simulink model "mbd_example_adc"  (R2022b)
settings: Solver=FixedStepDiscrete  StartTime=0.0  StopTime=10.0  RelTol=1e-3  EnableMultiTasking=on
PostLoadFcn:
  | run([bdroot '_init']);
InitFcn:
  | checkModelFolder(true); % Optional
  | run([bdroot '_init']);
values from neighbouring files (symbols this model uses):
  LED1_Hz = 2    [mbd_example_adc_init.m]
  LED2_Hz = 1    [mbd_example_adc_init.m]
  MBDDiag_Comm_Module = [2 3]    [mbd_example_adc_init.m]
  MBDDiag_Comm_Speed = [921600 921600]    [mbd_example_adc_init.m]
  MBDDiag_Comm_Type = [1 1]    [mbd_example_adc_init.m]
  T_s_LED1 = 1/LED1_Hz    (= 0.5)    [mbd_example_adc_init.m]
  T_s_LED2 = 1/LED2_Hz    (= 1)    [mbd_example_adc_init.m]
libraries: MbdLib_PortalDiag x26, MbdLib_Uart x15, MbdLib_SnapDiag x14, MbdLib_Digital x9, MbdLib_Analog x8, MbdLib_Timer x7, MbdLib_Sys x4, MbdLib_Pwm x2, MbdLib_Required x1
(part 1 of 2)
settings Model: Creator=KenYoshioka  LastModifiedBy=KenYoshioka
settings SolverCC: AutoInsertRateTranBlk=on
settings OptimizationCC: DefaultParameterBehavior=Inlined  DefaultUnderspecifiedDataType=single  EnhancedBackFolding=on  BooleansAsBitfields=on  PassReuseOutputArgsAs=Individual arguments  ZeroExternalMemoryAtStartup=off  ZeroInternalMemoryAtStartup=off  OptimizeBlockOrder=speed  DifferentSizesBufferReuse=on  EfficientTunableParamExpr=on
settings DebuggingCC: MultiTaskDSMMsg=none  ParameterTunabilityLossMsg=error
settings HardwareCC: ProdBitPerPointer=32  ProdBitPerSizeT=32  ProdBitPerPtrDiffT=32  ProdLargestAtomicInteger=Long  ProdLargestAtomicFloat=Double  ProdWordSize=32  ProdHWDeviceType=ARM Compatible->ARM Cortex-M
settings ModelReferenceCC: EnableRefExpFcnMdlSchedulingChecks=on  ModelReferenceNumInstancesAllowed=Single
settings SFSimCC: MATLABDynamicMemAlloc=off
settings RTWCC: Description=MBD Embedded Target STM32 Cortex M4 (real-time)  SystemTargetFile=MBD_STM32_stf.tlc  TemplateMakefile=MBD_STM32.tmf  Toolchain=arm-none-eabi - v10.3
settings CodeAppCC: ForceParamTrailComments=on  IgnoreCustomStorageClasses=off  MaxIdLength=255  OperatorAnnotations=on  SimulinkDataObjDesc=on  SFDataObjDesc=on  InsertBlockDesc=on
settings STFCustomTargetCC: MultiwordLength=256  IncludeMdlTerminateFcn=off  CombineOutputUpdateFcns=on  CombineSignalStateStructs=on  SuppressErrorStatus=on  ERTCustomFileBanners=on  SupportContinuousTime=off  RemoveResetFunc=on  MATLABClassNameForMDSCustomization=Simulink.SoftwareTarget.ERTCustomization  UseToolchainInfoCompliant=on  SystemTargetFile=MBD_STM32_stf.tlc
settings ERTTargetCC: ParMdlRefBuildCompliant=off  CompOptLevelCompliant=off  ConcurrentExecutionCompliant=off  IncludeMdlTerminateFcn=off  CombineSignalStateStructs=on  SuppressErrorStatus=on  SupportNonInlinedSFcns=on  ModelStepFunctionPrototypeControlCompliant=off  CPPClassGenCompliant=off  ExtModeStaticAllocSize=2000  InlinedParameterPlacement=NonHierarchical  ERTCustomFileTemplate=mbd_lib_interface.tlc  MaxLineWidth=110

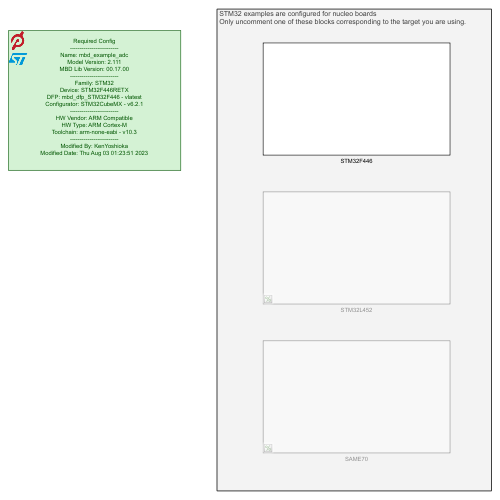
[thumbnail: Simulink's stored preview of the top-level diagram]
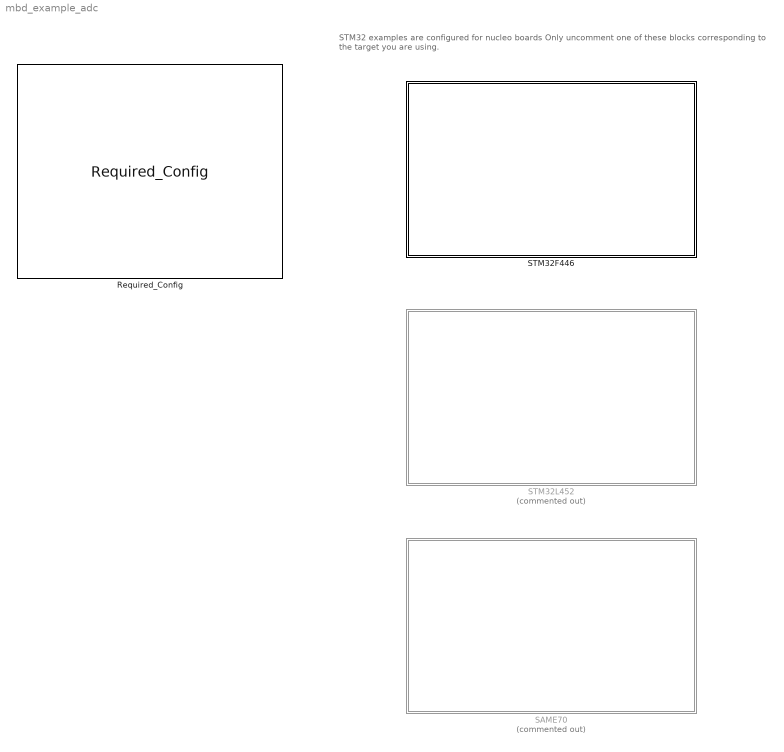
== system mbd_example_adc ==
  note: STM32 examples are configured for nucleo boards
      | Only uncomment one of these blocks corresponding to the target you are using.
  Required_Config : MbdLib_Required/Required_Config  Tag=MBD_Target_Info  Param_update=1
      settings: SourceProductName=Peloton Interface Library
  SAME70 : Subsystem  Commented=on
  STM32F446 : Subsystem
  STM32L452 : Subsystem  Commented=on

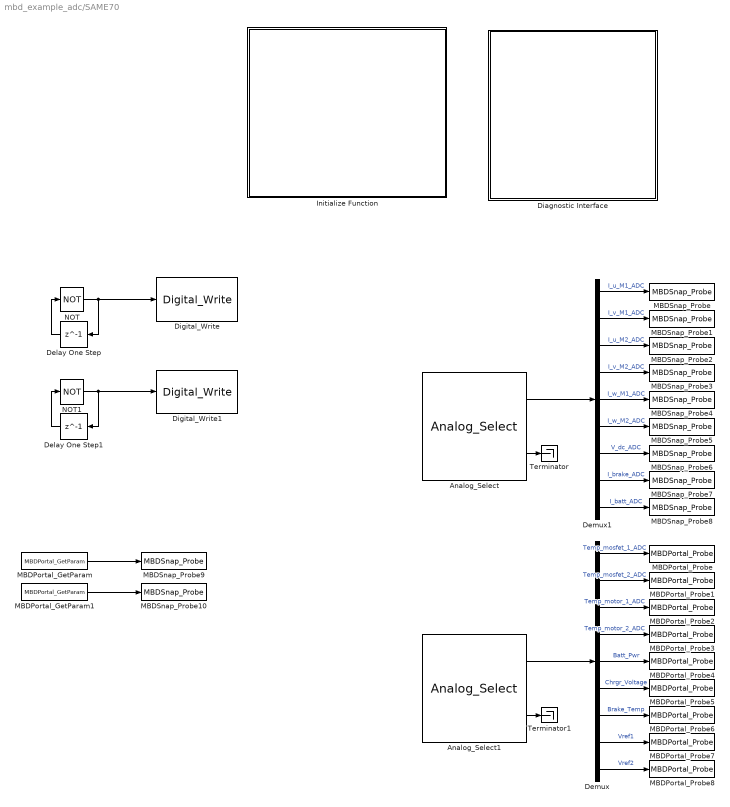
== system mbd_example_adc/SAME70 ==
  Analog_Select : MbdLib_Analog/Analog_Select  Param_triggerMode=No trigger  Param_module=0  Param_timeout=0  Param_outputNum=9  Param_module1=0  Param_index1=0  Param_module2=0  Param_index2=1  Param_module3=0  Param_index3=2  Param_module4=0  Param_index4=3  Param_module5=0  Param_index5=4  Param_module6=0  Param_index6=5  Param_module7=0  Param_index7=6  Param_module8=0  Param_index8=7  Param_module9=0  Param_index9=8  Param_module10=0  Param_index10=9  Param_module11=0  Param_index11=10  Param_module12=0  Param_index12=11  Param_sampleTime=T_s  Param_MBDUpdate=1
      settings: SourceProductName=Peloton Interface Library
  Analog_Select1 : MbdLib_Analog/Analog_Select  Param_triggerMode=No trigger  Param_module=0  Param_timeout=0  Param_outputNum=9  Param_module1=0  Param_index1=0  Param_module2=0  Param_index2=1  Param_module3=0  Param_index3=2  Param_module4=0  Param_index4=3  Param_module5=0  Param_index5=4  Param_module6=0  Param_index6=5  Param_module7=0  Param_index7=6  Param_module8=0  Param_index8=7  Param_module9=0  Param_index9=8  Param_module10=0  Param_index10=9  Param_module11=0  Param_index11=10  Param_module12=0  Param_index12=11  Param_sampleTime=T_s_COMM  Param_MBDUpdate=1
      settings: SourceProductName=Peloton Interface Library
  Delay One Step : Delay  DelayLength=1  SampleTime=LED1_Hz
  Delay One Step1 : Delay  DelayLength=1  SampleTime=LED2_Hz
  Demux : Demux  Outputs=9
  Demux1 : Demux  Outputs=9
  Diagnostic Interface : Subsystem
  Digital_Write : MbdLib_Digital/Digital_Write  Param_module=D  Param_ch=7  Param_sampleTime=-1
      settings: SourceProductName=Peloton Interface Library
  Digital_Write1 : MbdLib_Digital/Digital_Write  Param_module=D  Param_ch=8  Param_sampleTime=-1
      settings: SourceProductName=Peloton Interface Library
  Initialize Function : Subsystem  TreatAsAtomicUnit=on
  MBDPortal_GetParam : MbdLib_PortalDiag/MBDPortal_GetParam  Param_ParamName=start_snapshot  Param_ParamDefault=0  Param_ParamIndex=0  Param_ParamMax=MBDPortal_ParamNum
      settings: SourceProductName=Peloton Component Library
  MBDPortal_GetParam1 : MbdLib_PortalDiag/MBDPortal_GetParam  Param_ParamName=stop_snapshot  Param_ParamDefault=0  Param_ParamIndex=0  Param_ParamMax=MBDPortal_ParamNum
      settings: SourceProductName=Peloton Component Library
  MBDPortal_Probe : MbdLib_PortalDiag/MBDPortal_Probe  Param_SigNameInherited=on  Param_SigName=Temp_mosfet_1_ADC  Param_SigIndex=0  Param_SigMax=MBDPortal_SignalNum  Param_SampleTime=MBDPortal_CommonSampleRate
      settings: SourceProductName=Peloton Component Library
  MBDPortal_Probe1 : MbdLib_PortalDiag/MBDPortal_Probe  Param_SigNameInherited=on  Param_SigName=Temp_mosfet_2_ADC  Param_SigIndex=0  Param_SigMax=MBDPortal_SignalNum  Param_SampleTime=MBDPortal_CommonSampleRate
      settings: SourceProductName=Peloton Component Library
  MBDPortal_Probe2 : MbdLib_PortalDiag/MBDPortal_Probe  Param_SigNameInherited=on  Param_SigName=Temp_motor_1_ADC  Param_SigIndex=0  Param_SigMax=MBDPortal_SignalNum  Param_SampleTime=MBDPortal_CommonSampleRate
      settings: SourceProductName=Peloton Component Library
  MBDPortal_Probe3 : MbdLib_PortalDiag/MBDPortal_Probe  Param_SigNameInherited=on  Param_SigName=Temp_motor_2_ADC  Param_SigIndex=0  Param_SigMax=MBDPortal_SignalNum  Param_SampleTime=MBDPortal_CommonSampleRate
      settings: SourceProductName=Peloton Component Library
  MBDPortal_Probe4 : MbdLib_PortalDiag/MBDPortal_Probe  Param_SigNameInherited=on  Param_SigName=Batt_Pwr  Param_SigIndex=0  Param_SigMax=MBDPortal_SignalNum  Param_SampleTime=MBDPortal_CommonSampleRate
      settings: SourceProductName=Peloton Component Library
  MBDPortal_Probe5 : MbdLib_PortalDiag/MBDPortal_Probe  Param_SigNameInherited=on  Param_SigName=Chrgr_Voltage  Param_SigIndex=0  Param_SigMax=MBDPortal_SignalNum  Param_SampleTime=MBDPortal_CommonSampleRate
      settings: SourceProductName=Peloton Component Library
  MBDPortal_Probe6 : MbdLib_PortalDiag/MBDPortal_Probe  Param_SigNameInherited=on  Param_SigName=Brake_Temp  Param_SigIndex=0  Param_SigMax=MBDPortal_SignalNum  Param_SampleTime=MBDPortal_CommonSampleRate
      settings: SourceProductName=Peloton Component Library
  MBDPortal_Probe7 : MbdLib_PortalDiag/MBDPortal_Probe  Param_SigNameInherited=on  Param_SigName=Vref1  Param_SigIndex=0  Param_SigMax=MBDPortal_SignalNum  Param_SampleTime=MBDPortal_CommonSampleRate
      settings: SourceProductName=Peloton Component Library
  MBDPortal_Probe8 : MbdLib_PortalDiag/MBDPortal_Probe  Param_SigNameInherited=on  Param_SigName=Vref2  Param_SigIndex=0  Param_SigMax=MBDPortal_SignalNum  Param_SampleTime=MBDPortal_CommonSampleRate
      settings: SourceProductName=Peloton Component Library
  MBDSnap_Probe : MbdLib_SnapDiag/MBDSnap_Probe  Param_SigNameInherited=on  Param_SigName=I_u_M1_ADC  Param_SigIndex=0  Param_SigMax=MBDSnap_SignalNum  Param_StartEnable=off  Param_StartOpr=>  Param_StartThr=0  Param_StopEnable=off  Param_StopOpr=>  Param_StopThr=0  Param_StopPost=0  Param_SampleTime=MBDSnap_CommonSampleRate
      settings: SourceProductName=Peloton Component Library
  MBDSnap_Probe1 : MbdLib_SnapDiag/MBDSnap_Probe  Param_SigNameInherited=on  Param_SigName=I_v_M1_ADC  Param_SigIndex=0  Param_SigMax=MBDSnap_SignalNum  Param_StartEnable=off  Param_StartOpr=>  Param_StartThr=0  Param_StopEnable=off  Param_StopOpr=>  Param_StopThr=0  Param_StopPost=0  Param_SampleTime=MBDSnap_CommonSampleRate
      settings: SourceProductName=Peloton Component Library
  MBDSnap_Probe10 : MbdLib_SnapDiag/MBDSnap_Probe  Param_SigNameInherited=on  Param_SigName=stop_snapshot  Param_SigIndex=0  Param_SigMax=MBDSnap_SignalNum  Param_StartEnable=off  Param_StartOpr=>  Param_StartThr=0  Param_StopEnable=on  Param_StopOpr=>  Param_StopThr=0  Param_StopPost=0  Param_SampleTime=MBDSnap_CommonSampleRate
      settings: SourceProductName=Peloton Component Library
  MBDSnap_Probe2 : MbdLib_SnapDiag/MBDSnap_Probe  Param_SigNameInherited=on  Param_SigName=I_u_M2_ADC  Param_SigIndex=0  Param_SigMax=MBDSnap_SignalNum  Param_StartEnable=off  Param_StartOpr=>  Param_StartThr=0  Param_StopEnable=off  Param_StopOpr=>  Param_StopThr=0  Param_StopPost=0  Param_SampleTime=MBDSnap_CommonSampleRate
      settings: SourceProductName=Peloton Component Library
  MBDSnap_Probe3 : MbdLib_SnapDiag/MBDSnap_Probe  Param_SigNameInherited=on  Param_SigName=I_v_M2_ADC  Param_SigIndex=0  Param_SigMax=MBDSnap_SignalNum  Param_StartEnable=off  Param_StartOpr=>  Param_StartThr=0  Param_StopEnable=off  Param_StopOpr=>  Param_StopThr=0  Param_StopPost=0  Param_SampleTime=MBDSnap_CommonSampleRate
      settings: SourceProductName=Peloton Component Library
  MBDSnap_Probe4 : MbdLib_SnapDiag/MBDSnap_Probe  Param_SigNameInherited=on  Param_SigName=I_w_M1_ADC  Param_SigIndex=0  Param_SigMax=MBDSnap_SignalNum  Param_StartEnable=off  Param_StartOpr=>  Param_StartThr=0  Param_StopEnable=off  Param_StopOpr=>  Param_StopThr=0  Param_StopPost=0  Param_SampleTime=MBDSnap_CommonSampleRate
      settings: SourceProductName=Peloton Component Library
  MBDSnap_Probe5 : MbdLib_SnapDiag/MBDSnap_Probe  Param_SigNameInherited=on  Param_SigName=I_w_M2_ADC  Param_SigIndex=0  Param_SigMax=MBDSnap_SignalNum  Param_StartEnable=off  Param_StartOpr=>  Param_StartThr=0  Param_StopEnable=off  Param_StopOpr=>  Param_StopThr=0  Param_StopPost=0  Param_SampleTime=MBDSnap_CommonSampleRate
      settings: SourceProductName=Peloton Component Library
  MBDSnap_Probe6 : MbdLib_SnapDiag/MBDSnap_Probe  Param_SigNameInherited=on  Param_SigName=V_dc_ADC  Param_SigIndex=0  Param_SigMax=MBDSnap_SignalNum  Param_StartEnable=off  Param_StartOpr=>  Param_StartThr=0  Param_StopEnable=off  Param_StopOpr=>  Param_StopThr=0  Param_StopPost=0  Param_SampleTime=MBDSnap_CommonSampleRate
      settings: SourceProductName=Peloton Component Library
  MBDSnap_Probe7 : MbdLib_SnapDiag/MBDSnap_Probe  Param_SigNameInherited=on  Param_SigName=I_brake_ADC  Param_SigIndex=0  Param_SigMax=MBDSnap_SignalNum  Param_StartEnable=off  Param_StartOpr=>  Param_StartThr=0  Param_StopEnable=off  Param_StopOpr=>  Param_StopThr=0  Param_StopPost=0  Param_SampleTime=MBDSnap_CommonSampleRate
      settings: SourceProductName=Peloton Component Library
  MBDSnap_Probe8 : MbdLib_SnapDiag/MBDSnap_Probe  Param_SigNameInherited=on  Param_SigName=I_batt_ADC  Param_SigIndex=0  Param_SigMax=MBDSnap_SignalNum  Param_StartEnable=off  Param_StartOpr=>  Param_StartThr=0  Param_StopEnable=off  Param_StopOpr=>  Param_StopThr=0  Param_StopPost=0  Param_SampleTime=MBDSnap_CommonSampleRate
      settings: SourceProductName=Peloton Component Library
  MBDSnap_Probe9 : MbdLib_SnapDiag/MBDSnap_Probe  Param_SigNameInherited=on  Param_SigName=start_snapshot  Param_SigIndex=0  Param_SigMax=MBDSnap_SignalNum  Param_StartEnable=on  Param_StartOpr=>  Param_StartThr=0  Param_StopEnable=off  Param_StopOpr=>  Param_StopThr=0  Param_StopPost=0  Param_SampleTime=MBDSnap_CommonSampleRate
      settings: SourceProductName=Peloton Component Library
  NOT : Logic  Operator=NOT  IconShape=distinctive  AllPortsSameDT=off  OutDataTypeStr=boolean
  NOT1 : Logic  Operator=NOT  IconShape=distinctive  AllPortsSameDT=off  OutDataTypeStr=boolean
  Terminator : Terminator
  Terminator1 : Terminator
  wires:
  Analog_Select1/1 -> Demux/1
  MBDPortal_GetParam/1 -> MBDSnap_Probe9/1
  MBDPortal_GetParam1/1 -> MBDSnap_Probe10/1
  Demux1/3 -> MBDSnap_Probe2/1  "I_u_M2_ADC"
  Demux/9 -> MBDPortal_Probe8/1  "Vref2"
  Demux/7 -> MBDPortal_Probe6/1  "Brake_Temp"
  Demux/2 -> MBDPortal_Probe1/1  "Temp_mosfet_2_ADC"
  Demux/8 -> MBDPortal_Probe7/1  "Vref1"
  Delay One Step/1 -> NOT/1
  Demux/4 -> MBDPortal_Probe3/1  "Temp_motor_2_ADC"
  Demux1/5 -> MBDSnap_Probe4/1  "I_w_M1_ADC"
  Demux1/4 -> MBDSnap_Probe3/1  "I_v_M2_ADC"
  Demux/6 -> MBDPortal_Probe5/1  "Chrgr_Voltage"
  Demux1/6 -> MBDSnap_Probe5/1  "I_w_M2_ADC"
  Demux1/1 -> MBDSnap_Probe/1  "I_u_M1_ADC"
  Demux/3 -> MBDPortal_Probe2/1  "Temp_motor_1_ADC"
  Demux1/7 -> MBDSnap_Probe6/1  "V_dc_ADC"
  Demux1/8 -> MBDSnap_Probe7/1  "I_brake_ADC"
  Demux/5 -> MBDPortal_Probe4/1  "Batt_Pwr"
  Demux1/9 -> MBDSnap_Probe8/1  "I_batt_ADC"
  Demux1/2 -> MBDSnap_Probe1/1  "I_v_M1_ADC"
  Analog_Select/1 -> Demux1/1
  NOT/1 -> Digital_Write/1, Delay One Step/1
  Demux/1 -> MBDPortal_Probe/1  "Temp_mosfet_1_ADC"
  NOT1/1 -> Digital_Write1/1, Delay One Step1/1
  Delay One Step1/1 -> NOT1/1
  Analog_Select/2 -> Terminator/1
  Analog_Select1/2 -> Terminator1/1

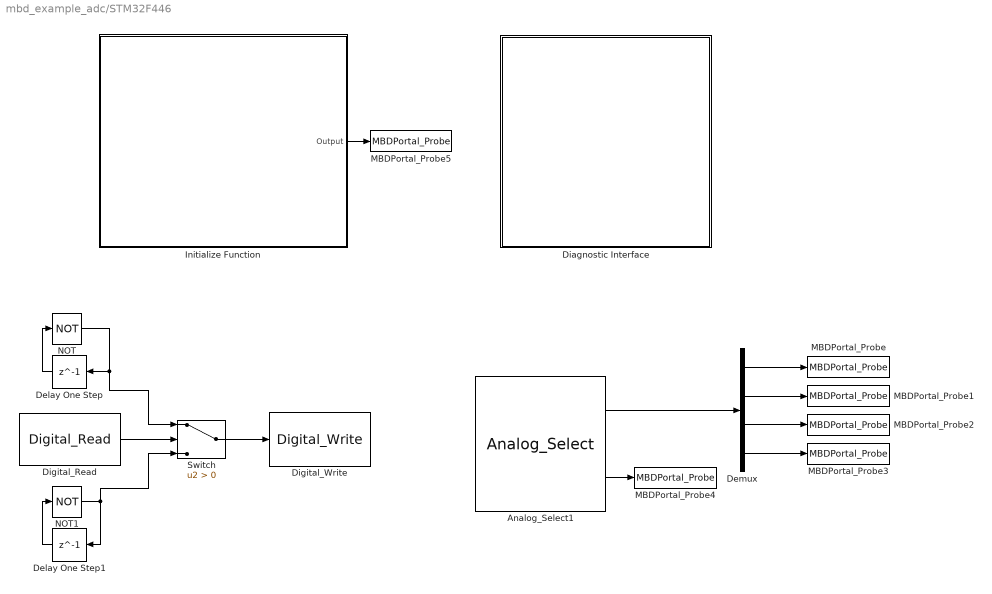
== system mbd_example_adc/STM32F446 ==
  Analog_Select1 : MbdLib_Analog/Analog_Select  Param_triggerMode=Trigger and block until acquisition  Param_module=1  Param_timeout=0  Param_outputNum=4  Param_module1=1  Param_index1=0  Param_module2=1  Param_index2=1  Param_module3=1  Param_index3=2  Param_module4=1  Param_index4=3  Param_module5=1  Param_index5=4  Param_module6=1  Param_index6=5  Param_module7=1  Param_index7=6  Param_module8=1  Param_index8=7  Param_module9=1  Param_index9=8  Param_module10=0  Param_index10=9  Param_module11=0  Param_index11=10  Param_module12=0  Param_index12=11  Param_sampleTime=T_s_COMM  Param_MBDUpdate=1
      settings: SourceProductName=Peloton Interface Library
  Delay One Step : Delay  DelayLength=1  SampleTime=T_s_LED1
  Delay One Step1 : Delay  DelayLength=1  SampleTime=T_s_LED2
  Demux : Demux
  Diagnostic Interface : Subsystem
  Digital_Read : MbdLib_Digital/Digital_Read  Param_module=C  Param_ch=13  Param_sampleTime=-1  Sim_invert=off  Sim_out=0
      settings: SourceProductName=Peloton Interface Library
  Digital_Write : MbdLib_Digital/Digital_Write  Param_module=C  Param_ch=10  Param_sampleTime=-1
      settings: SourceProductName=Peloton Interface Library
  Initialize Function : Subsystem  TreatAsAtomicUnit=on
  MBDPortal_Probe : MbdLib_PortalDiag/MBDPortal_Probe  Param_SigNameInherited=off  Param_SigName=ADC1_IN1  Param_SigIndex=0  Param_SigMax=MBDPortal_SignalNum  Param_SampleTime=MBDPortal_CommonSampleRate
      settings: SourceProductName=Peloton Component Library
  MBDPortal_Probe1 : MbdLib_PortalDiag/MBDPortal_Probe  Param_SigNameInherited=off  Param_SigName=ADC1_IN2  Param_SigIndex=0  Param_SigMax=MBDPortal_SignalNum  Param_SampleTime=MBDPortal_CommonSampleRate
      settings: SourceProductName=Peloton Component Library
  MBDPortal_Probe2 : MbdLib_PortalDiag/MBDPortal_Probe  Param_SigNameInherited=on  Param_SigName=ADC1_IN3  Param_SigIndex=0  Param_SigMax=MBDPortal_SignalNum  Param_SampleTime=MBDPortal_CommonSampleRate
      settings: SourceProductName=Peloton Component Library
  MBDPortal_Probe3 : MbdLib_PortalDiag/MBDPortal_Probe  Param_SigNameInherited=on  Param_SigName=ADC1_IN4  Param_SigIndex=0  Param_SigMax=MBDPortal_SignalNum  Param_SampleTime=MBDPortal_CommonSampleRate
      settings: SourceProductName=Peloton Component Library
  MBDPortal_Probe4 : MbdLib_PortalDiag/MBDPortal_Probe  Param_SigNameInherited=on  Param_SigName=ADC_read_status  Param_SigIndex=0  Param_SigMax=MBDPortal_SignalNum  Param_SampleTime=MBDPortal_CommonSampleRate
      settings: SourceProductName=Peloton Component Library
  MBDPortal_Probe5 : MbdLib_PortalDiag/MBDPortal_Probe  Param_SigNameInherited=on  Param_SigName=ADC_config_status  Param_SigIndex=0  Param_SigMax=MBDPortal_SignalNum  Param_SampleTime=MBDPortal_CommonSampleRate
      settings: SourceProductName=Peloton Component Library
  NOT : Logic  Operator=NOT  IconShape=distinctive  AllPortsSameDT=off  OutDataTypeStr=boolean
  NOT1 : Logic  Operator=NOT  IconShape=distinctive  AllPortsSameDT=off  OutDataTypeStr=boolean
  Switch : Switch  Criteria=u2 > Threshold  SaturateOnIntegerOverflow=off  InputSameDT=off
  wires:
  NOT/1 -> Switch/1, Delay One Step/1
  NOT1/1 -> Switch/3, Delay One Step1/1
  Delay One Step1/1 -> NOT1/1
  Switch/1 -> Digital_Write/1
  Digital_Read/1 -> Switch/2
  Delay One Step/1 -> NOT/1
  Analog_Select1/2 -> MBDPortal_Probe4/1
  Demux/3 -> MBDPortal_Probe2/1
  Analog_Select1/1 -> Demux/1
  Demux/2 -> MBDPortal_Probe1/1
  Demux/4 -> MBDPortal_Probe3/1
  Demux/1 -> MBDPortal_Probe/1
  Initialize Function/1(Output) -> MBDPortal_Probe5/1

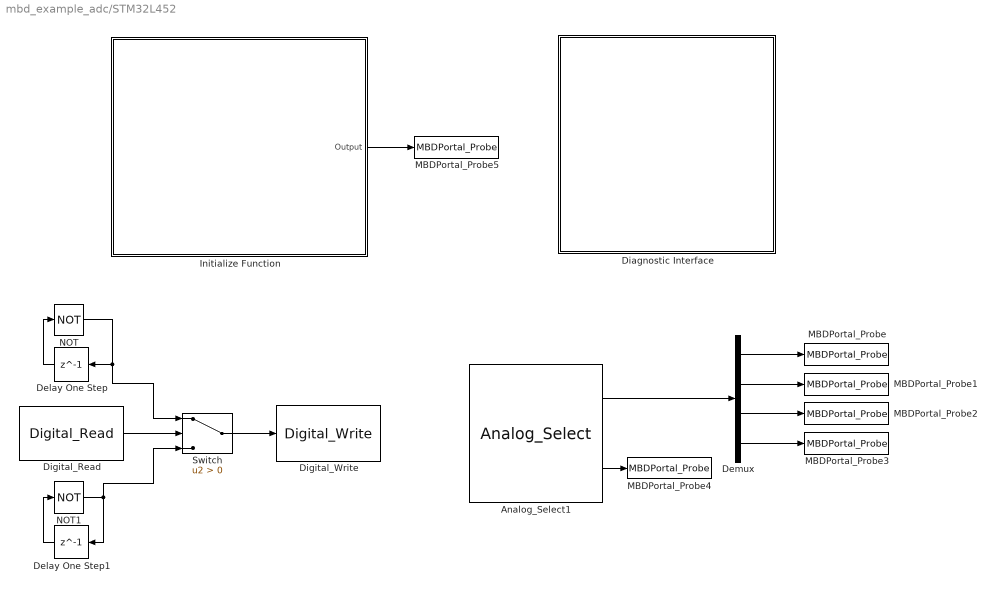
== system mbd_example_adc/STM32L452 ==
  Analog_Select1 : MbdLib_Analog/Analog_Select  Param_triggerMode=No trigger  Param_module=1  Param_timeout=0  Param_outputNum=4  Param_module1=1  Param_index1=0  Param_module2=1  Param_index2=1  Param_module3=1  Param_index3=2  Param_module4=1  Param_index4=3  Param_module5=1  Param_index5=4  Param_module6=1  Param_index6=5  Param_module7=1  Param_index7=6  Param_module8=1  Param_index8=7  Param_module9=1  Param_index9=8  Param_module10=0  Param_index10=9  Param_module11=0  Param_index11=10  Param_module12=0  Param_index12=11  Param_sampleTime=T_s_COMM  Param_MBDUpdate=1
      settings: SourceProductName=Peloton Interface Library
  Delay One Step : Delay  DelayLength=1  SampleTime=T_s_LED1
  Delay One Step1 : Delay  DelayLength=1  SampleTime=T_s_LED2
  Demux : Demux
  Diagnostic Interface : Subsystem
  Digital_Read : MbdLib_Digital/Digital_Read  Param_module=C  Param_ch=13  Param_sampleTime=-1  Sim_invert=off  Sim_out=0
      settings: SourceProductName=Peloton Interface Library
  Digital_Write : MbdLib_Digital/Digital_Write  Param_module=C  Param_ch=10  Param_sampleTime=-1
      settings: SourceProductName=Peloton Interface Library
  Initialize Function : Subsystem  TreatAsAtomicUnit=on
  MBDPortal_Probe : MbdLib_PortalDiag/MBDPortal_Probe  Param_SigNameInherited=off  Param_SigName=ADC1_IN1  Param_SigIndex=0  Param_SigMax=MBDPortal_SignalNum  Param_SampleTime=MBDPortal_CommonSampleRate
      settings: SourceProductName=Peloton Component Library
  MBDPortal_Probe1 : MbdLib_PortalDiag/MBDPortal_Probe  Param_SigNameInherited=off  Param_SigName=ADC1_IN2  Param_SigIndex=0  Param_SigMax=MBDPortal_SignalNum  Param_SampleTime=MBDPortal_CommonSampleRate
      settings: SourceProductName=Peloton Component Library
  MBDPortal_Probe2 : MbdLib_PortalDiag/MBDPortal_Probe  Param_SigNameInherited=on  Param_SigName=ADC1_IN3  Param_SigIndex=0  Param_SigMax=MBDPortal_SignalNum  Param_SampleTime=MBDPortal_CommonSampleRate
      settings: SourceProductName=Peloton Component Library
  MBDPortal_Probe3 : MbdLib_PortalDiag/MBDPortal_Probe  Param_SigNameInherited=on  Param_SigName=ADC1_IN4  Param_SigIndex=0  Param_SigMax=MBDPortal_SignalNum  Param_SampleTime=MBDPortal_CommonSampleRate
      settings: SourceProductName=Peloton Component Library
  MBDPortal_Probe4 : MbdLib_PortalDiag/MBDPortal_Probe  Param_SigNameInherited=on  Param_SigName=ADC_read_status  Param_SigIndex=0  Param_SigMax=MBDPortal_SignalNum  Param_SampleTime=MBDPortal_CommonSampleRate
      settings: SourceProductName=Peloton Component Library
  MBDPortal_Probe5 : MbdLib_PortalDiag/MBDPortal_Probe  Param_SigNameInherited=on  Param_SigName=ADC_config_status  Param_SigIndex=0  Param_SigMax=MBDPortal_SignalNum  Param_SampleTime=MBDPortal_CommonSampleRate
      settings: SourceProductName=Peloton Component Library
  NOT : Logic  Operator=NOT  IconShape=distinctive  AllPortsSameDT=off  OutDataTypeStr=boolean
  NOT1 : Logic  Operator=NOT  IconShape=distinctive  AllPortsSameDT=off  OutDataTypeStr=boolean
  Switch : Switch  Criteria=u2 > Threshold  SaturateOnIntegerOverflow=off  InputSameDT=off
  wires:
  Analog_Select1/1 -> Demux/1
  Demux/2 -> MBDPortal_Probe1/1
  Demux/4 -> MBDPortal_Probe3/1
  Demux/3 -> MBDPortal_Probe2/1
  Demux/1 -> MBDPortal_Probe/1
  NOT1/1 -> Switch/3, Delay One Step1/1
  NOT/1 -> Switch/1, Delay One Step/1
  Switch/1 -> Digital_Write/1
  Digital_Read/1 -> Switch/2
  Delay One Step1/1 -> NOT1/1
  Delay One Step/1 -> NOT/1
  Analog_Select1/2 -> MBDPortal_Probe4/1
  Initialize Function/1(Output) -> MBDPortal_Probe5/1

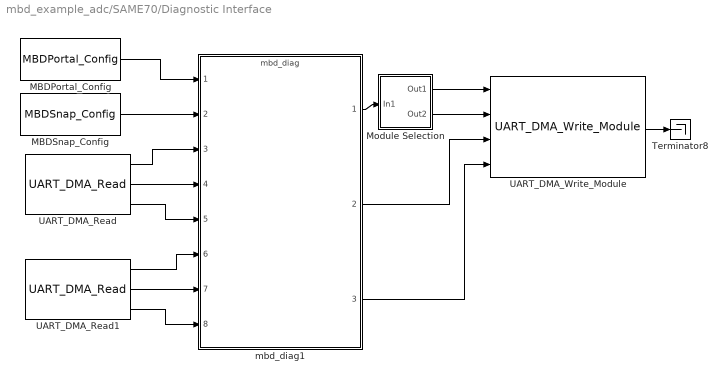
== system mbd_example_adc/SAME70/Diagnostic Interface ==
  MBDPortal_Config : MbdLib_PortalDiag/MBDPortal_Config  Param_SigMax=MBDPortal_SignalNum  Param_ParamMax=MBDPortal_ParamNum
      settings: SourceProductName=Peloton Component Library
  MBDSnap_Config : MbdLib_SnapDiag/MBDSnap_Config  Priority=-5000  Param_enableAll=on  Param_SampleTime=T_s_COMM  Param_SigMax=MBDSnap_SignalNum
      settings: SourceProductName=Peloton Component Library
  Module Selection : Subsystem
  Terminator8 : Terminator
  UART_DMA_Read : MbdLib_Uart/UART_DMA_Read  Tag=TAG_UART_DMA  Param_module=MBDDiag_Comm_Module(1)  Param_type=USART  Param_readLim=100  Param_sampleTime=T_s_COMM
      settings: SourceProductName=Peloton Interface Library
  UART_DMA_Read1 : MbdLib_Uart/UART_DMA_Read  Tag=TAG_UART_DMA  Param_module=MBDDiag_Comm_Module(2)  Param_type=USART  Param_readLim=100  Param_sampleTime=T_s_COMM
      settings: SourceProductName=Peloton Interface Library
  UART_DMA_Write_Module : MbdLib_Uart/UART_DMA_Write_Module  Param_instanceNum=2  Param_module1=MBDDiag_Comm_Module(1)  Param_type1=USART  Param_module2=MBDDiag_Comm_Module(2)  Param_type2=USART  Param_module3=0  Param_type3=UART  Param_module4=0  Param_type4=UART  Param_sampleTime=-1  Sim_status=0
      settings: SourceProductName=Peloton Interface Library
  mbd_diag1 : ModelReference  ModelNameDialog=mbd_diag.slx  SimulationMode=Normal  ModelReferenceVersion=2.294  SimulationMode=Normal
  wires:
  Module Selection/2(Out2) -> UART_DMA_Write_Module/2
  UART_DMA_Read1/2 -> mbd_diag1/7
  UART_DMA_Read/1 -> mbd_diag1/3
  UART_DMA_Write_Module/1 -> Terminator8/1
  mbd_diag1/1 -> Module Selection/1(In1)
  MBDPortal_Config/1 -> mbd_diag1/1
  mbd_diag1/3 -> UART_DMA_Write_Module/4
  MBDSnap_Config/1 -> mbd_diag1/2
  mbd_diag1/2 -> UART_DMA_Write_Module/3
  UART_DMA_Read/2 -> mbd_diag1/4
  Module Selection/1(Out1) -> UART_DMA_Write_Module/1
  UART_DMA_Read1/1 -> mbd_diag1/6
  UART_DMA_Read1/3 -> mbd_diag1/8
  UART_DMA_Read/3 -> mbd_diag1/5

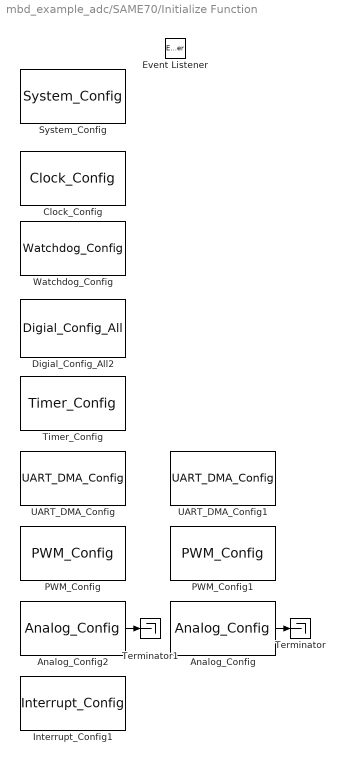
== system mbd_example_adc/SAME70/Initialize Function ==
  Analog_Config : MbdLib_Analog/Analog_Config  Priority=70  Param_module=1  Param_step=-1  Param_preScaler=3  Param_startUpTime=4  Param_signMode=2  Param_resolution=0  Param_hwTrigEn=on  Param_hwTrigSel=4  Param_swTrigEn=off  Param_gainEnable=on  Param_channels={ '0', 'on', 'B', '1', '0', '0', '512', 'off', 'on'; '1', 'on', 'C', '13', '1', '0', '512', 'off', 'on'; '2', 'on', 'C', '15', '3', '0', '512', 'off', 'off'; '3', 'off', 'A', '0', 'disable', '0', '0', 'off', 'off'; '4', 'on', 'C', '29', '2', '0', '512', 'off', 'on'; '5', 'on', 'C', '30', '4', '0', '512', 'off', 'on'; '6', 'on', 'C', '31', 'disable', '0', '512', 'off', 'off'; '7', 'on', 'C', '26', 'disable', '0', '512', 'off', 'off'; '8', 'off', 'A', '0', 'disable', '0', '0', 'off', 'off'; '9', 'off', 'A', '0', 'disable', '0', '0', 'off', 'off'; '10', 'on', 'E', '3', 'disable', '0', '512', 'off', 'off'; '11', 'on', 'E', '0', 'disable', '0', '512', 'off', 'off' }  Param_priority=70  Param_sampleTime=-1
      settings: AttributesFormatString=priority=%<priority>  SourceProductName=Peloton Interface Library
  Analog_Config2 : MbdLib_Analog/Analog_Config  Priority=70  Param_module=0  Param_step=-1  Param_preScaler=3  Param_startUpTime=4  Param_signMode=2  Param_resolution=0  Param_hwTrigEn=on  Param_hwTrigSel=4  Param_swTrigEn=off  Param_gainEnable=on  Param_channels={ '0', 'on', 'D', '30', '0', '0', '512', 'off', 'on'; '1', 'on', 'A', '21', '1', '0', '512', 'off', 'on'; '2', 'on', 'B', '3', '2', '0', '512', 'on', 'on'; '3', 'on', 'E', '5', '3', '0', '512', 'off', 'on'; '4', 'on', 'E', '4', '4', '0', '512', 'off', 'on'; '5', 'off', 'A', '0', 'disable', '0', '0', 'off', 'off'; '6', 'on', 'A', '17', 'disable', '0', '512', 'off', 'off'; '7', 'on', 'A', '18', 'disable', '0', '512', 'off', 'off'; '8', 'on', 'A', '19', 'disable', '0', '512', 'off', 'off'; '9', 'on', 'A', '20', 'disable', '0', '512', 'off', 'off'; '10', 'on', 'B', '0', 'disable', '0', '512', 'off', 'off'; '11', 'off', 'A', '0', 'disable', '0', '0', 'off', 'off' }  Param_priority=70  Param_sampleTime=-1
      settings: AttributesFormatString=priority=%<priority>  SourceProductName=Peloton Interface Library
  Clock_Config : MbdLib_Sys/Clock_Config  Priority=10  Param_frequency=Peripheral_Clock_Hz  Param_priority=10  Param_sampleTime=-1
      settings: AttributesFormatString=priority=%<priority>  SourceProductName=Peloton Interface Library
  Digial_Config_All2 : MbdLib_Digital/Digial_Config_All  Priority=30  Param_channels={ 'A', '0', 'off', '0 : input', '0 : low', '0 : none', '0 : none', '0 : low', '0 : low'; 'A', '1', 'off', '0 : input', '0 : low', '0 : none', '0 : none', '0 : low', '0 : low'; 'A', '2', 'off', '0 : input', '0 : low', '0 : none', '0 : none', '0 : low', '0 : low'; 'A', '3', 'off', '0 : input', '0 : low', '0 : none', '0 : none', '0 : low', '0 : low'; 'A', '4', 'off', '0 : input', '0 : low', '0 : none', '0 : none', '0 : low', '0 : low'; 'A', '5', 'off', '0 : input', '0 : low', '0 : none', '0 : none', '0 : low', '0 : low'; 'A', '6', 'off', '0 : input', '0 : low', '0 : none', '0 : none', '0 : low', '0 : low'; 'A', '7', 'off', '0 : input', '0 : low', '0 : none', '0 : none', '0 : low', '0 : low'; 'A', '8', 'off', '0 : input', '0 : low', '0 : none', '0 : none', '0 : low', '0 : low'; 'A', '9', 'off', '0 : input', '0 : low', '0 : none', '0 : none', '0 : low', '0 : low'; 'A', '10', 'off', '0 : input', '0 : low', '0 : none', '0 : none', '0 : low', '0 : low'; 'A', '11', 'off', '0 : input', '0 : low', '0 : none', '0 : none', '0 : low', '0 : low'; 'A', '12', 'off', '0 : input', '0 : low', '0 : none', '0 : none', '0 : low', '0 : low'; 'A', '13', 'off', '0 : input', '0 : low', '0 : none', '0 : none', '0 : low', '0 : low'; 'A', '14', 'off', '0 : input', '0 : low', '0 : none', '0 : none', '0 : low', '0 : low'; 'A', '15', 'off', '0 : input', '0 : low', '0 : none', '0 : none', '0 : low', '0 : low'; 'A', '16', 'off', '0 : input', '0 : low', '0 : none', '0 : none', '0 : low', '0 : low'; 'A', '17', 'off', '0 : input', '0 : low', '0 : none', '0 : none', '0 : low', '0 : low'; 'A', '18', 'off', '0 : input', '0 : low', '0 : none', '0 : none', '0 : low', '0 : low'; 'A', '19', 'off', '0 : input', '0 : low', '0 : none', '0 : none', '0 : low', '0 : low'; 'A', '20', 'off', '0 : input', '0 : low', '0 : none', '0 : none', '0 : low', '0 : low'; 'A', '21', 'off', '0 : input', '0 : low', '0 : none', '0 : none', '0 : low', '0 : low'; 'A', '22', 'off', '0 : input', '0 : low', '0 : none', '0 : none', '0 : low', '0 : low'; 'A', '23', 'off', '0 : input', '0 : low', '0 : none', '0 : none', '0 : low', '0 : low'; 'A', '24', 'off', '0 : input', '0 : low', '0 : none', '0 : none', '0 : low', '0 : low'; 'A', '25', 'off', '0 : input', '0 : low', '0 : none', '0 : none', '0 : low', '0 : low'; 'A', '26', 'off', '0 : input', '0 : low', '0 : none', '0 : none', '0 : low', '0 : low'; 'A', '27', 'off', '0 : input', '0 : low', '0 : none', '0 : none', '0 : low', '0 : low'; 'A', '28', 'off', '0 : input', '0 : low', '0 : none', '0 : none', '0 : low', '0 : low'; 'A', '29', 'off', '0 : input', '0 : low', '0 : none', '0 : none', '0 : low', '0 : low'; 'A', '30', 'off', '0 : input', '0 : low', '0 : none', '0 : none', '0 : low', '0 : low'; 'A', '31', 'off', '0 : input', '0 : low', '0 : none', '0 : none', '0 : low', '0 : low'; 'B', '0', 'off', '0 : input', '0 : low', '0 : none', '0 : none', '0 : low', '0 : low'; 'B', '1', 'off', '0 : input', '0 : low', '0 : none', '0 : none', '0 : low', '0 : low'; 'B', '2', 'off', '0 : input', '0 : low', '0 : none', '0 : none', '0 : low', '0 : low'; 'B', '3', 'off', '0 : input', '0 : low', '0 : none', '0 : none', '0 : low', '0 : low'; 'B', '4', 'off', '0 : input', '0 : low', '0 : none', '0 : none', '0 : low', '0 : low'; 'B', '5', 'off', '0 : input', '0 : low', '0 : none', '0 : none', '0 : low', '0 : low'; 'B', '6', 'off', '0 : input', '0 : low', '0 : none', '0 : none', '0 : low', '0 : low'; 'B', '7', 'off', '0 : input', '0 : low', '0 : none', '0 : none', '0 : low', '0 : low'; 'B', '8', 'off', '0 : input', '0 : low', '0 : none', '0 : none', '0 : low', '0 : low'; 'B', '9', 'off', '0 : input', '0 : low', '0 : none', '0 : none', '0 : low', '0 : low'; 'B', '10', 'off', '0 : input', '0 : low', '0 : none', '0 : none', '0 : low', '0 : low'; 'B', '11', 'off', '0 : input', '0 : low', '0 : none', '0 : none', '0 : low', '0 : low'; 'B', '12', 'off', '0 : input', '0 : low', '0 : none', '0 : none', '0 : low', '0 : low'; 'B', '13', 'off', '0 : input', '0 : low', '0 : none', '0 : none', '0 : low', '0 : low'; 'C', '0', 'off', '0 : input', '0 : low', '0 : none', '0 : none', '0 : low', '0 : low'; 'C', '1', 'off', '0 : input', '0 : low', '0 : none', '0 : none', '0 : low', '0 : low'; 'C', '2', 'off', '0 : input', '0 : low', '0 : none', '0 : none', '0 : low', '0 : low'; 'C', '3', 'off', '0 : input', '0 : low', '0 : none', '0 : none', '0 : low', '0 : low'; 'C', '4', 'off', '0 : input', '0 : low', '0 : none', '0 : none', '0 : low', '0 : low'; 'C', '5', 'off', '0 : input', '0 : low', '0 : none', '0 : none', '0 : low', '0 : low'; 'C', '6', 'off', '0 : input', '0 : low', '0 : none', '0 : none', '0 : low', '0 : low'; 'C', '7', 'off', '0 : input', '0 : low', '0 : none', '0 : none', '0 : low', '0 : low'; 'C', '8', 'off', '0 : input', '0 : low', '0 : none', '0 : none', '0 : low', '0 : low'; 'C', '9', 'off', '0 : input', '0 : low', '0 : none', '0 : none', '0 : low', '0 : low'; 'C', '10', 'off', '0 : input', '0 : low', '0 : none', '0 : none', '0 : low', '0 : low'; 'C', '11', 'off', '0 : input', '0 : low', '0 : none', '0 : none', '0 : low', '0 : low'; 'C', '12', 'off', '0 : input', '0 : low', '0 : none', '0 : none', '0 : low', '0 : low'; 'C', '13', 'off', '0 : input', '0 : low', '0 : none', '0 : none', '0 : low', '0 : low'; 'C', '14', 'off', '0 : input', '0 : low', '0 : none', '0 : none', '0 : low', '0 : low'; 'C', '15', 'off', '0 : input', '0 : low', '0 : none', '0 : none', '0 : low', '0 : low'; 'C', '16', 'off', '0 : input', '0 : low', '0 : none', '0 : none', '0 : low', '0 : low'; 'C', '17', 'off', '0 : input', '0 : low', '0 : none', '0 : none', '0 : low', '0 : low'; 'C', '18', 'off', '0 : input', '0 : low', '0 : none', '0 : none', '0 : low', '0 : low'; 'C', '19', 'off', '0 : input', '0 : low', '0 : none', '0 : none', '0 : low', '0 : low'; 'C', '20', 'off', '0 : input', '0 : low', '0 : none', '0 : none', '0 : low', '0 : low'; 'C', '21', 'off', '0 : input', '0 : low', '0 : none', '0 : none', '0 : low', '0 : low'; 'C', '22', 'off', '0 : input', '0 : low', '0 : none', '0 : none', '0 : low', '0 : low'; 'C', '23', 'off', '0 : input', '0 : low', '0 : none', '0 : none', '0 : low', '0 : low'; 'C', '24', 'off', '0 : input', '0 : low', '0 : none', '0 : none', '0 : low', '0 : low'; 'C', '25', 'off', '0 : input', '0 : low', '0 : none', '0 : none', '0 : low', '0 : low'; 'C', '26', 'off', '0 : input', '0 : low', '0 : none', '0 : none', '0 : low', '0 : low'; 'C', '27', 'off', '0 : input', '0 : low', '0 : none', '0 : none', '0 : low', '0 : low'; 'C', '28', 'off', '0 : input', '0 : low', '0 : none', '0 : none', '0 : low', '0 : low'; 'C', '29', 'off', '0 : input', '0 : low', '0 : none', '0 : none', '0 : low', '0 : low'; 'C', '30', 'off', '0 : input', '0 : low', '0 : none', '0 : none', '0 : low', '0 : low'; 'C', '31', 'off', '0 : input', '0 : low', '0 : none', '0 : none', '0 : low', '0 : low'; 'D', '0', 'off', '0 : input', '0 : low', '0 : none', '0 : none', '0 : low', '0 : low'; 'D', '1', 'off', '0 : input', '0 : low', '0 : none', '0 : none', '0 : low', '0 : low'; 'D', '2', 'off', '0 : input', '0 : low', '0 : none', '0 : none', '0 : low', '0 : low'; 'D', '3', 'off', '0 : input', '0 : low', '0 : none', '0 : none', '0 : low', '0 : low'; 'D', '4', 'off', '0 : input', '0 : low', '0 : none', '0 : none', '0 : low', '0 : low'; 'D', '5', 'off', '0 : input', '0 : low', '0 : none', '0 : none', '0 : low', '0 : low'; 'D', '6', 'off', '0 : input', '0 : low', '0 : none', '0 : none', '0 : low', '0 : low'; 'D', '7', 'on', '1 : output', '0 : low', '0 : none', '0 : none', '0 : low', '0 : low'; 'D', '8', 'on', '1 : output', '0 : low', '0 : none', '0 : none', '0 : low', '0 : low'; 'D', '9', 'on', '1 : output', '0 : low', '0 : none', '0 : none', '0 : low', '0 : low'; 'D', '10', 'off', '0 : input', '0 : low', '0 : none', '0 : none', '0 : low', '0 : low'; 'D', '11', 'off', '0 : input', '0 : low', '0 : none', '0 : none', '0 : low', '0 : low'; 'D', '12', 'off', '0 : input', '0 : low', '0 : none', '0 : none', '0 : low', '0 : low'; 'D', '13', 'off', '0 : input', '0 : low', '0 : none', '0 : none', '0 : low', '0 : low'; 'D', '14', 'off', '0 : input', '0 : low', '0 : none', '0 : none', '0 : low', '0 : low'; 'D', '15', 'off', '0 : input', '0 : low', '0 : none', '0 : none', '0 : low', '0 : low'; 'D', '16', 'off', '0 : input', '0 : low', '0 : none', '0 : none', '0 : low', '0 : low'; 'D', '17', 'off', '0 : input', '0 : low', '0 : none', '0 : none', '0 : low', '0 : low'; 'D', '18', 'off', '0 : input', '0 : low', '0 : none', '0 : none', '0 : low', '0 : low'; 'D', '19', 'off', '0 : input', '0 : low', '0 : none', '0 : none', '0 : low', '0 : low'; 'D', '20', 'off', '0 : input', '0 : low', '0 : none', '0 : none', '0 : low', '0 : low'; 'D', '21', 'off', '0 : input', '0 : low', '0 : none', '0 : none', '0 : low', '0 : low'; 'D', '22', 'off', '0 : input', '0 : low', '0 : none', '0 : none', '0 : low', '0 : low'; 'D', '23', 'off', '0 : input', '0 : low', '0 : none', '0 : none', '0 : low', '0 : low'; 'D', '24', 'off', '0 : input', '0 : low', '0 : none', '0 : none', '0 : low', '0 : low'; 'D', '25', 'off', '0 : input', '0 : low', '0 : none', '0 : none', '0 : low', '0 : low'; 'D', '26', 'off', '0 : input', '0 : low', '0 : none', '0 : none', '0 : low', '0 : low'; 'D', '27', 'off', '0 : input', '0 : low', '0 : none', '0 : none', '0 : low', '0 : low'; 'D', '28', 'off', '0 : input', '0 : low', '0 : none', '0 : none', '0 : low', '0 : low'; 'D', '29', 'off', '0 : input', '0 : low', '0 : none', '0 : none', '0 : low', '0 : low'; 'D', '30', 'off', '0 : input', '0 : low', '0 : none', '0 : none', '0 : low', '0 : low'; 'D', '31', 'off', '0 : input', '0 : low', '0 : none', '0 : none', '0 : low', '0 : low'; 'E', '0', 'off', '0 : input', '0 : low', '0 : none', '0 : none', '0 : low', '0 : low'; 'E', '1', 'off', '0 : input', '0 : low', '0 : none', '0 : none', '0 : low', '0 : low'; 'E', '2', 'off', '0 : input', '0 : low', '0 : none', '0 : none', '0 : low', '0 : low'; 'E', '3', 'off', '0 : input', '0 : low', '0 : none', '0 : none', '0 : low', '0 : low'; 'E', '4', 'off', '0 : input', '0 : low', '0 : none', '0 : none', '0 : low', '0 : low'; 'E', '5', 'off', '0 : input', '0 : low', '0 : none', '0 : none', '0 : low', '0 : low' }  Param_priority=30  Param_sampleTime=-1
      settings: AttributesFormatString=priority=%<priority>  SourceProductName=Peloton Interface Library
  Event Listener : EventListener  DisableCoverage=on  EventName=reset
  Interrupt_Config1 : MbdLib_Sys/Interrupt_Config  Priority=120  Param_priority=120  Param_sampleTime=-1
      settings: AttributesFormatString=priority=%<priority>  SourceProductName=Peloton Interface Library
  PWM_Config : MbdLib_Pwm/PWM_Config  Priority=60  Param_module=0  Param_clksrc=0  Param_period=PWM_period_cycles  Param_channels={ '0', 'on', 'PWM_period_cycles/2', '120', 'on'; '1', 'on', 'PWM_period_cycles/2', '120', 'on'; '2', 'on', 'PWM_period_cycles/2', '120', 'on'; '3', 'off', '0', '0', 'off' }  Param_priority=60  Param_sampleTime=-1
      settings: AttributesFormatString=priority=%<priority>  SourceProductName=Peloton Interface Library
  PWM_Config1 : MbdLib_Pwm/PWM_Config  Priority=60  Param_module=1  Param_clksrc=0  Param_period=PWM_period_cycles  Param_channels={ '0', 'on', 'PWM_period_cycles/2', '120', 'on'; '1', 'on', 'PWM_period_cycles/2', '120', 'on'; '2', 'on', 'PWM_period_cycles/2', '120', 'on'; '3', 'on', 'PWM_period_cycles/2', '120', 'off' }  Param_priority=60  Param_sampleTime=-1
      settings: AttributesFormatString=priority=%<priority>  SourceProductName=Peloton Interface Library
  System_Config : MbdLib_Sys/System_Config  Priority=0  Param_priority=0  Param_sampleTime=-1
      settings: AttributesFormatString=priority=%<priority>  SourceProductName=Peloton Interface Library
  Terminator : Terminator
  Terminator1 : Terminator
  Timer_Config : MbdLib_Timer/Timer_Config  Priority=40  Param_update=1  Param_module=2  Param_step=1  Param_period=Comm_period_cycles  Param_divider=0  Param_step0=1  Param_clksrc0=1  Param_period0=Comm_period_cycles  Param_divider0=0  Param_step1=2  Param_clksrc1=2  Param_period1=LED1_period_cycles  Param_divider1=0  Param_step2=3  Param_clksrc2=2  Param_period2=LED2_period_cycles  Param_divider2=0  Param_priority=40  Param_sampleTime=-1
      settings: AttributesFormatString=priority=%<priority>  SourceProductName=Peloton Interface Library
  UART_DMA_Config : MbdLib_Uart/UART_DMA_Config  Priority=50  Param_module=0  Param_type=UART  Param_speed=921600  Param_dataBits=8  Param_stopBits=0.5  Param_parity=None  Param_priority=50  Param_sampleTime=-1
      settings: AttributesFormatString=priority=%<priority>  SourceProductName=Peloton Interface Library
  UART_DMA_Config1 : MbdLib_Uart/UART_DMA_Config  Priority=50  Param_module=1  Param_type=UART  Param_speed=921600  Param_dataBits=8  Param_stopBits=0.5  Param_parity=None  Param_priority=50  Param_sampleTime=-1
      settings: AttributesFormatString=priority=%<priority>  SourceProductName=Peloton Interface Library
  Watchdog_Config : MbdLib_Sys/Watchdog_Config  Priority=20  Param_enable=off  Param_priority=20  Param_sampleTime=-1
      settings: AttributesFormatString=priority=%<priority>  SourceProductName=Peloton Interface Library
  wires:
  Analog_Config/1 -> Terminator/1
  Analog_Config2/1 -> Terminator1/1

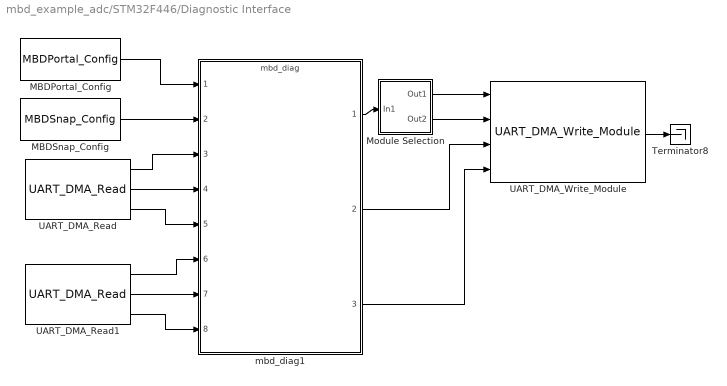
== system mbd_example_adc/STM32F446/Diagnostic Interface ==
  MBDPortal_Config : MbdLib_PortalDiag/MBDPortal_Config  Param_SigMax=MBDPortal_SignalNum  Param_ParamMax=MBDPortal_ParamNum
      settings: SourceProductName=Peloton Component Library
  MBDSnap_Config : MbdLib_SnapDiag/MBDSnap_Config  Priority=-5000  Param_enableAll=on  Param_SampleTime=T_s_COMM  Param_SigMax=MBDSnap_SignalNum
      settings: SourceProductName=Peloton Component Library
  Module Selection : Subsystem
  Terminator8 : Terminator
  UART_DMA_Read : MbdLib_Uart/UART_DMA_Read  Tag=TAG_UART_DMA  Param_module=MBDDiag_Comm_Module(1)  Param_type=USART  Param_readLim=100  Param_sampleTime=T_s_COMM
      settings: SourceProductName=Peloton Interface Library
  UART_DMA_Read1 : MbdLib_Uart/UART_DMA_Read  Tag=TAG_UART_DMA  Param_module=MBDDiag_Comm_Module(2)  Param_type=USART  Param_readLim=100  Param_sampleTime=T_s_COMM
      settings: SourceProductName=Peloton Interface Library
  UART_DMA_Write_Module : MbdLib_Uart/UART_DMA_Write_Module  Param_instanceNum=2  Param_module1=MBDDiag_Comm_Module(1)  Param_type1=USART  Param_module2=MBDDiag_Comm_Module(2)  Param_type2=USART  Param_module3=0  Param_type3=UART  Param_module4=0  Param_type4=UART  Param_sampleTime=-1  Sim_status=0
      settings: SourceProductName=Peloton Interface Library
  mbd_diag1 : ModelReference  ModelNameDialog=mbd_diag.slx  SimulationMode=Normal  ModelReferenceVersion=2.298  SimulationMode=Normal
  wires:
  Module Selection/2(Out2) -> UART_DMA_Write_Module/2
  UART_DMA_Read1/2 -> mbd_diag1/7
  UART_DMA_Read/1 -> mbd_diag1/3
  UART_DMA_Write_Module/1 -> Terminator8/1
  mbd_diag1/1 -> Module Selection/1(In1)
  MBDPortal_Config/1 -> mbd_diag1/1
  mbd_diag1/3 -> UART_DMA_Write_Module/4
  MBDSnap_Config/1 -> mbd_diag1/2
  mbd_diag1/2 -> UART_DMA_Write_Module/3
  UART_DMA_Read/2 -> mbd_diag1/4
  Module Selection/1(Out1) -> UART_DMA_Write_Module/1
  UART_DMA_Read1/1 -> mbd_diag1/6
  UART_DMA_Read/3 -> mbd_diag1/5
  UART_DMA_Read1/3 -> mbd_diag1/8
